simulink model "BFSK"  (R2023b)
settings: Solver=VariableStepAuto  StartTime=0.0  StopTime=10  RelTol=1e-3
settings Model: Creator=mluser  LastModifiedBy=mluser

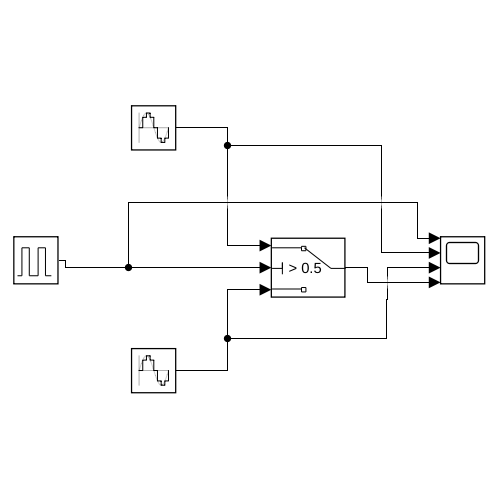
[thumbnail: Simulink's stored preview of the top-level diagram]
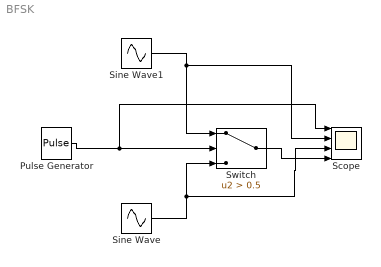
== system BFSK ==
  Pulse Generator : DiscretePulseGenerator  PulseType=Time based  PulseWidth=50
  Scope : Scope  NumInputPorts=4
  Sine Wave : Sin  Frequency=2*pi*4  SampleTime=0.01
  Sine Wave1 : Sin  Frequency=2*pi*10  SampleTime=0.01
  Switch : Switch  Criteria=u2 > Threshold  Threshold=0.5  SaturateOnIntegerOverflow=off  InputSameDT=off
  wires:
  Pulse Generator/1 -> Scope/1, Switch/2
  Sine Wave/1 -> Scope/3, Switch/3
  Sine Wave1/1 -> Scope/2, Switch/1
  Switch/1 -> Scope/4
